simulink model "MSMS"  (Simulink 7.7)
settings: Solver=ode45  StartTime=0.0  StopTime=50  RelTol=1e-3
settings Model: Creator=cadaverProject  LastModifiedBy=cadaverProject

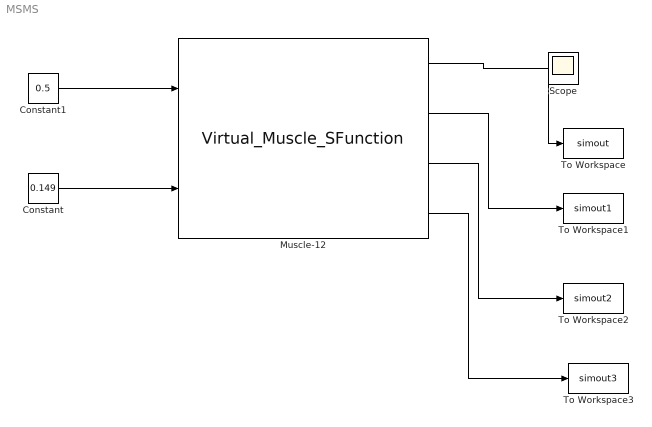
== system MSMS ==
  Constant : Constant  Value=0.149
  Constant1 : Constant  Value=0.5
  Muscle-12 : S-Function  FunctionName=Virtual_Muscle_SFunction  Parameters=TOFMUSFIB SARCLEN SPTEN VISC C1 K1 LR1 C2 K2 LR2 CT KT LRT RRANK V05 F05 FMIN FMAX FLOMEGA FLBETA FLRHO VMAX CV0 CV1 AV0 AV1 AV2 BV AF NF0 NF1 TL TF1 TF2 TF3 TF4 AS1 AS2 TS CY VY TY CH0 CH1 CH2 CH3 RTYPE ADDPORTS MMASS FASCL0 TENDL0T LPATH UR NUMOFUNITS FPCSA UPCSA APPORTMTD GEOPCSA  EnableBusSupport=off  mask{RTYPE=2, ADDPORTS=[1 0 0], FASCL0=9.891476996222012, TENDL0T=4.945738498111007, LPATH=17.804658593199623, MMASS=100.0, UR=0.8, SPTEN=31.8, VISC=0.01, SARCLEN=2.7, C1=23.0, K1=0.046, LR1=1.17, C2=-0.02, K2=-18.7, LR2=0.79, CT=27.8, KT=0.0047, LRT=0.964, TOFMUSFIB=2, FPCSA=[0.5 0.5], NUMOFUNITS=[1 1], APPORTMTD=2, GEOPCSA=0.0010, UPCSA=[0.5 0.5], RRANK=[2 3], V05=[-1.2123 -2.5547], F05=[20.0 34.0], FMIN=[0.5 0.5], FMAX=[2.0 2.0], FLOMEGA=[1.1244 0.74633], FLBETA=[2.3 1.55], FLRHO=[1.62 2.12], VMAX=[-7.88 -9.1516], CV0=[5.88 -5.7], CV1=[0.0 9.18], AV0=[-4.7 -1.53], AV1=[8.41 0.0], AV2=[-5.31 0.0], BV=[0.34936 0.68637], AF=[0.56 0.56], NF0=[2.11 2.11], NF1=[5.0 3.31], TL=[0.088 0.088], TF1=[34.2833 20.57], TF2=[22.6667 13.6], TF3=[47.0333 28.22], TF4=[25.2167 15.13], AS1=[1.0 1.76], AS2=[1.0 0.96], TS=[1.0 43.0], CY=[0.35 0.0], VY=[0.1 1.0], TY=[200.0 1.0], CH0=[1.01 1.6866], CH1=[0.38 0.38], CH2=[0.43 0.43], CH3=[0.31 0.51769]}
      mask prompts: RTYPE "Recruitment Type (1-Natural Units, 2-Natural Lumped, 3-Intramuscular FES)"; ADDPORTS "Additional Outputs"; FASCL0 "Optimal Fascicle Length (cm)"; TENDL0T "Optimal Tendon Length (cm)"; LPATH "Maximum Path Length (cm)"; MMASS "Muscle Mass (g)"; UR "Maximum Recruitment Excitation (Ur)"; SPTEN "Specific Tension (N/cm2)"; VISC "Viscosity (part of FPE1)"; SARCLEN "Optimal sarcomere length (um)"; C1 "C1 (FPE1)"; K1 "K1 (FPE1)"; LR1 "LR1 (FPE1)"; C2 "C2 (FPE2)"; K2 "K2 (FPE2)"; LR2 "LR2 (FPE2)"; CT "CT (FSE)"; KT "KT (FSE)"; LRT "LRT (FSE)"; TOFMUSFIB "Number of Fiber Types"; FPCSA "Fractional PCSA for Each Muscle Fiber Type"; NUMOFUNITS "Number of motor units in each muscle fiber type"; APPORTMTD "Apportion Method (1-Manual, 2-Default, 3-Geometric, 4-Equal)"; GEOPCSA "Fractional increase in PCSA for Geometric Apportion Method"; UPCSA "PCSA for Each Motor Unit (Manual changes effective only for Apportion Method 1)"; RRANK "Recruitment Rank"; V05 "V0.5 (L0/S)"; F05 "f0.5 (pps)"; FMIN "fmin (f0.5)"; FMAX "fmax (f0.5)"; FLOMEGA "FL_omega"; FLBETA "FL_beta"; FLRHO "FL_rho"
      mask Display: port_label('input', 1,'Excitation (0-1)'); port_label('input', 2,'MT path length (m)'); port_label('output',1,'Force (N)'); port_label('output',2,'Force (F0)'); port_label('output',3,'Lce (L0)');port_label('output',4,'Vce (L0/s)');disp('VM');
  Scope : Scope
  To Workspace : ToWorkspace  VariableName=simout  SampleTime=-1  SaveFormat=Structure
  To Workspace1 : ToWorkspace  VariableName=simout1  SampleTime=-1  SaveFormat=Structure
  To Workspace2 : ToWorkspace  VariableName=simout2  SampleTime=-1  SaveFormat=Structure
  To Workspace3 : ToWorkspace  VariableName=simout3  SampleTime=-1  SaveFormat=Structure
  wires:
  Muscle-12/1 -> To Workspace/1
  Constant1/1 -> Muscle-12/1
  Constant/1 -> Muscle-12/2
  Muscle-12/2 -> To Workspace1/1
  Muscle-12/3 -> To Workspace2/1
  Muscle-12/4 -> To Workspace3/1
